simulink model "fkine_test1"  (R2018b)
settings: Solver=FixedStepAuto  StartTime=0.0  StopTime=30  FixedStep=0.01  RelTol=1e-3
InitFcn:
  | runfirst
values from neighbouring files (symbols this model uses):
  bL = 22    [runfirst.m]
  bWb = 15.5    [runfirst.m]
  bWs = 13.5    [runfirst.m]
  d1 = 0    [runfirst.m]
  d2 = 0    [runfirst.m]
  L1 = 3.4    [runfirst.m]
  L2 = 9.5    [runfirst.m]
  L3 = 14.2    [runfirst.m]
settings Model: Creator=skakd  LastModifiedBy=skakd

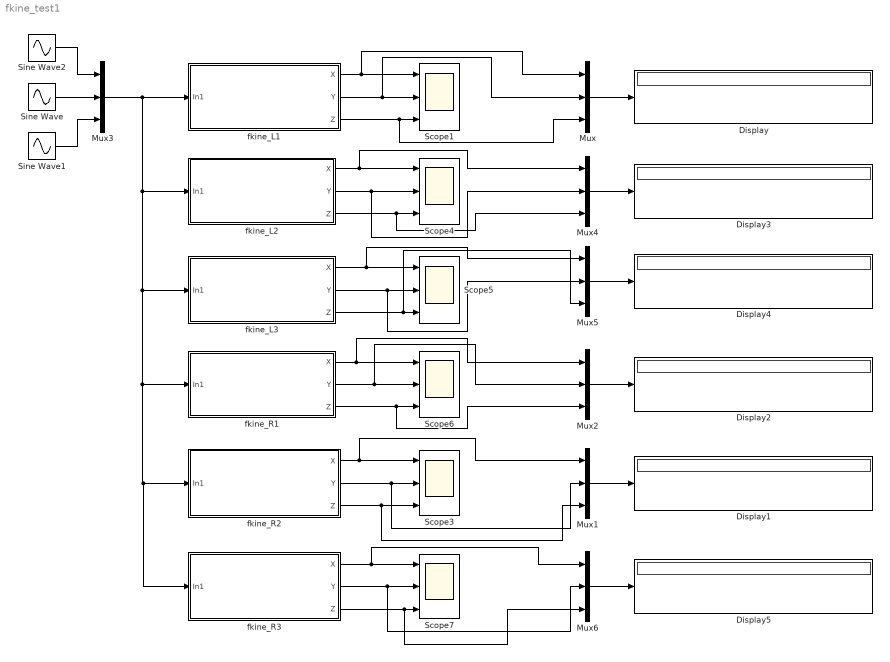
== system fkine_test1 ==
  Display{,1..5} (6 alike) : Display
  Mux{,1..6} (7 alike) : Mux  Inputs=3
  Scope{1,3..7} (6 alike) : Scope  NumInputPorts=3
  Sine Wave : Sin  Amplitude=10  SampleTime=0
  Sine Wave1 : Sin  Amplitude=2.4  Frequency=1.7  SampleTime=0
  Sine Wave2 : Sin  Amplitude=3  Frequency=3.5  SampleTime=0
  fkine_L1 : Subsystem
  fkine_L2 : Subsystem
  fkine_L3 : Subsystem
  fkine_R1 : Subsystem
  fkine_R2 : Subsystem
  fkine_R3 : Subsystem
  wires:
  Sine Wave/1 -> Mux3/2
  Sine Wave1/1 -> Mux3/3
  Sine Wave2/1 -> Mux3/1
  Mux3/1 -> fkine_R3/1(In1), fkine_R2/1(In1), fkine_R1/1(In1), fkine_L3/1(In1), fkine_L2/1(In1), fkine_L1/1(In1)
  fkine_R2/1(X) -> Mux1/1, Scope3/1
  fkine_R2/2(Y) -> Mux1/2, Scope3/2
  fkine_R2/3(Z) -> Mux1/3, Scope3/3
  fkine_L1/1(X) -> Mux/1, Scope1/1
  fkine_L1/2(Y) -> Mux/2, Scope1/2
  fkine_L1/3(Z) -> Mux/3, Scope1/3
  fkine_L2/1(X) -> Mux4/1, Scope4/1
  fkine_L2/2(Y) -> Mux4/2, Scope4/2
  fkine_L2/3(Z) -> Mux4/3, Scope4/3
  fkine_L3/1(X) -> Mux5/1, Scope5/1
  fkine_L3/2(Y) -> Mux5/2, Scope5/2
  fkine_L3/3(Z) -> Mux5/3, Scope5/3
  fkine_R1/1(X) -> Mux2/1, Scope6/1
  fkine_R1/2(Y) -> Mux2/2, Scope6/2
  fkine_R1/3(Z) -> Mux2/3, Scope6/3
  fkine_R3/1(X) -> Mux6/1, Scope7/1
  fkine_R3/2(Y) -> Mux6/2, Scope7/2
  fkine_R3/3(Z) -> Mux6/3, Scope7/3
  Mux/1 -> Display/1
  Mux1/1 -> Display1/1
  Mux2/1 -> Display2/1
  Mux4/1 -> Display3/1
  Mux5/1 -> Display4/1
  Mux6/1 -> Display5/1

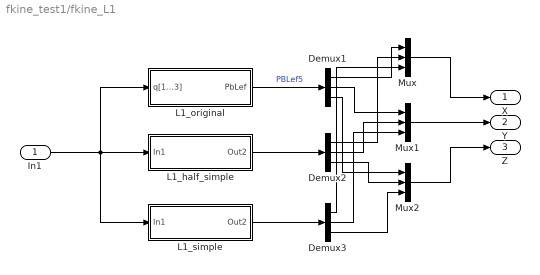
== system fkine_test1/fkine_L1 ==
  In1 : Inport
  Demux1 : Demux  Outputs=3
  Demux2 : Demux  Outputs=3
  Demux3 : Demux  Outputs=3
  L1_half_simple : Subsystem
  L1_original : Subsystem
  L1_simple : Subsystem
  Mux : Mux  Inputs=3
  Mux1 : Mux  Inputs=3
  Mux2 : Mux  Inputs=3
  X : Outport
  Y : Outport  Port=2
  Z : Outport  Port=3
  wires:
  Demux3/2 -> Mux1/3
  L1_original/1(PbLef) -> Demux1/1  "PBLef5"
  Demux3/1 -> Mux/3
  Demux1/1 -> Mux/1
  Demux2/2 -> Mux1/2
  Demux1/3 -> Mux2/1
  Mux2/1 -> Z/1
  Demux1/2 -> Mux1/1
  L1_simple/1(Out2) -> Demux3/1
  Demux2/3 -> Mux2/2
  L1_half_simple/1(Out2) -> Demux2/1
  In1/1 -> L1_simple/1(In1), L1_half_simple/1(In1), L1_original/1(q[1...3])
  Demux2/1 -> Mux/2
  Demux3/3 -> Mux2/3
  Mux/1 -> X/1
  Mux1/1 -> Y/1

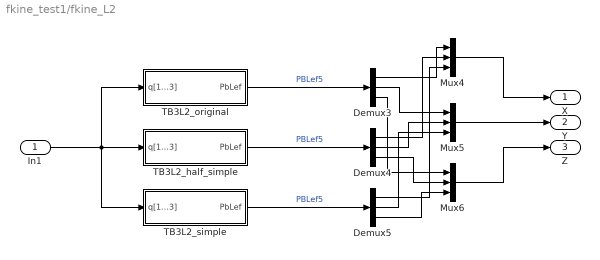
== system fkine_test1/fkine_L2 ==
  In1 : Inport
  Demux3 : Demux  Outputs=3
  Demux4 : Demux  Outputs=3
  Demux5 : Demux  Outputs=3
  Mux4 : Mux  Inputs=3
  Mux5 : Mux  Inputs=3
  Mux6 : Mux  Inputs=3
  TB3L2_half_simple : Subsystem
  TB3L2_original : Subsystem
  TB3L2_simple : Subsystem
  X : Outport
  Y : Outport  Port=2
  Z : Outport  Port=3
  wires:
  Demux4/1 -> Mux4/2
  In1/1 -> TB3L2_half_simple/1(q[1...3]), TB3L2_simple/1(q[1...3]), TB3L2_original/1(q[1...3])
  Demux3/1 -> Mux4/1
  Demux4/2 -> Mux5/2
  TB3L2_half_simple/1(PbLef) -> Demux4/1  "PBLef5"
  Demux5/1 -> Mux4/3
  Demux3/2 -> Mux5/1
  Demux3/3 -> Mux6/1
  Demux5/2 -> Mux5/3
  Demux4/3 -> Mux6/2
  TB3L2_original/1(PbLef) -> Demux3/1  "PBLef5"
  TB3L2_simple/1(PbLef) -> Demux5/1  "PBLef5"
  Demux5/3 -> Mux6/3
  Mux6/1 -> Z/1
  Mux5/1 -> Y/1
  Mux4/1 -> X/1

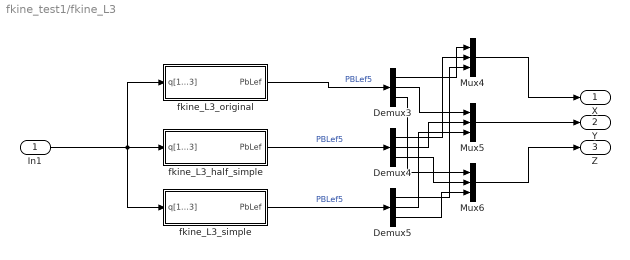
== system fkine_test1/fkine_L3 ==
  In1 : Inport
  Demux3 : Demux  Outputs=3
  Demux4 : Demux  Outputs=3
  Demux5 : Demux  Outputs=3
  Mux4 : Mux  Inputs=3
  Mux5 : Mux  Inputs=3
  Mux6 : Mux  Inputs=3
  fkine_L3_half_simple : Subsystem
  fkine_L3_original : Subsystem
  fkine_L3_simple : Subsystem
  X : Outport
  Y : Outport  Port=2
  Z : Outport  Port=3
  wires:
  Demux3/3 -> Mux6/1
  fkine_L3_original/1(PbLef) -> Demux3/1  "PBLef5"
  In1/1 -> fkine_L3_original/1(q[1...3]), fkine_L3_simple/1(q[1...3]), fkine_L3_half_simple/1(q[1...3])
  Demux3/2 -> Mux5/1
  Demux4/3 -> Mux6/2
  Demux5/1 -> Mux4/3
  fkine_L3_simple/1(PbLef) -> Demux5/1  "PBLef5"
  Demux5/3 -> Mux6/3
  Demux3/1 -> Mux4/1
  Demux5/2 -> Mux5/3
  Mux6/1 -> Z/1
  Demux4/1 -> Mux4/2
  Mux5/1 -> Y/1
  Demux4/2 -> Mux5/2
  Mux4/1 -> X/1
  fkine_L3_half_simple/1(PbLef) -> Demux4/1  "PBLef5"

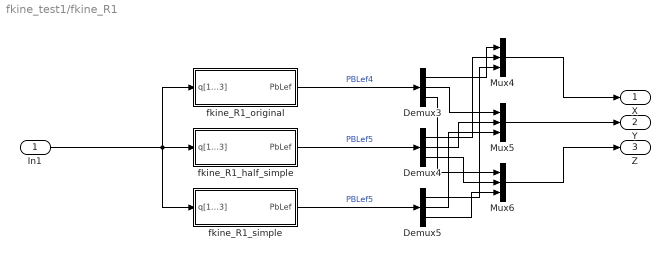
== system fkine_test1/fkine_R1 ==
  In1 : Inport
  Demux3 : Demux  Outputs=3
  Demux4 : Demux  Outputs=3
  Demux5 : Demux  Outputs=3
  Mux4 : Mux  Inputs=3
  Mux5 : Mux  Inputs=3
  Mux6 : Mux  Inputs=3
  fkine_R1_half_simple : Subsystem
  fkine_R1_original : Subsystem
  fkine_R1_simple : Subsystem
  X : Outport
  Y : Outport  Port=2
  Z : Outport  Port=3
  wires:
  Demux3/3 -> Mux6/1
  Demux3/1 -> Mux4/1
  In1/1 -> fkine_R1_simple/1(q[1...3]), fkine_R1_original/1(q[1...3]), fkine_R1_half_simple/1(q[1...3])
  fkine_R1_half_simple/1(PbLef) -> Demux4/1  "PBLef5"
  fkine_R1_simple/1(PbLef) -> Demux5/1  "PBLef5"
  Demux4/1 -> Mux4/2
  Demux5/3 -> Mux6/3
  Demux5/2 -> Mux5/3
  Demux5/1 -> Mux4/3
  Demux4/3 -> Mux6/2
  Demux3/2 -> Mux5/1
  Mux4/1 -> X/1
  Demux4/2 -> Mux5/2
  fkine_R1_original/1(PbLef) -> Demux3/1  "PBLef4"
  Mux6/1 -> Z/1
  Mux5/1 -> Y/1

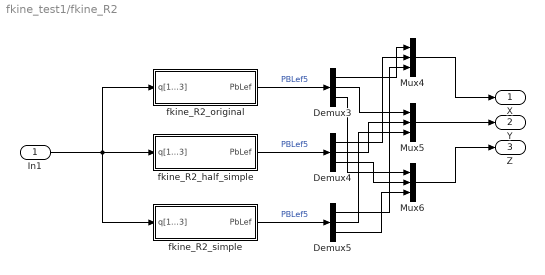
== system fkine_test1/fkine_R2 ==
  In1 : Inport
  Demux3 : Demux  Outputs=3
  Demux4 : Demux  Outputs=3
  Demux5 : Demux  Outputs=3
  Mux4 : Mux  Inputs=3
  Mux5 : Mux  Inputs=3
  Mux6 : Mux  Inputs=3
  fkine_R2_half_simple : Subsystem
  fkine_R2_original : Subsystem
  fkine_R2_simple : Subsystem
  X : Outport
  Y : Outport  Port=2
  Z : Outport  Port=3
  wires:
  Demux3/2 -> Mux5/1
  fkine_R2_half_simple/1(PbLef) -> Demux4/1  "PBLef5"
  Demux4/1 -> Mux4/2
  In1/1 -> fkine_R2_half_simple/1(q[1...3]), fkine_R2_simple/1(q[1...3]), fkine_R2_original/1(q[1...3])
  Demux4/2 -> Mux5/2
  fkine_R2_simple/1(PbLef) -> Demux5/1  "PBLef5"
  Demux5/1 -> Mux4/3
  Demux5/2 -> Mux5/3
  Demux5/3 -> Mux6/3
  Demux3/1 -> Mux4/1
  Demux3/3 -> Mux6/1
  Demux4/3 -> Mux6/2
  fkine_R2_original/1(PbLef) -> Demux3/1  "PBLef5"
  Mux6/1 -> Z/1
  Mux4/1 -> X/1
  Mux5/1 -> Y/1

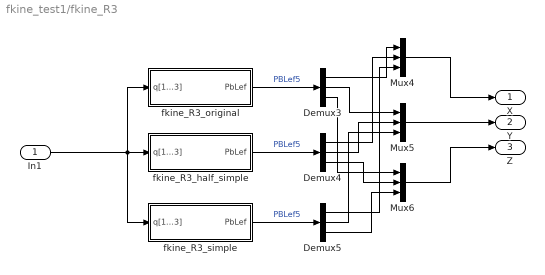
== system fkine_test1/fkine_R3 ==
  In1 : Inport
  Demux3 : Demux  Outputs=3
  Demux4 : Demux  Outputs=3
  Demux5 : Demux  Outputs=3
  Mux4 : Mux  Inputs=3
  Mux5 : Mux  Inputs=3
  Mux6 : Mux  Inputs=3
  fkine_R3_half_simple : Subsystem
  fkine_R3_original : Subsystem
  fkine_R3_simple : Subsystem
  X : Outport
  Y : Outport  Port=2
  Z : Outport  Port=3
  wires:
  Demux4/3 -> Mux6/2
  In1/1 -> fkine_R3_original/1(q[1...3]), fkine_R3_simple/1(q[1...3]), fkine_R3_half_simple/1(q[1...3])
  Demux3/3 -> Mux6/1
  fkine_R3_simple/1(PbLef) -> Demux5/1  "PBLef5"
  fkine_R3_original/1(PbLef) -> Demux3/1  "PBLef5"
  Demux4/1 -> Mux4/2
  Demux3/1 -> Mux4/1
  Demux5/2 -> Mux5/3
  Mux6/1 -> Z/1
  Demux4/2 -> Mux5/2
  Demux5/3 -> Mux6/3
  Demux5/1 -> Mux4/3
  Demux3/2 -> Mux5/1
  fkine_R3_half_simple/1(PbLef) -> Demux4/1  "PBLef5"
  Mux4/1 -> X/1
  Mux5/1 -> Y/1

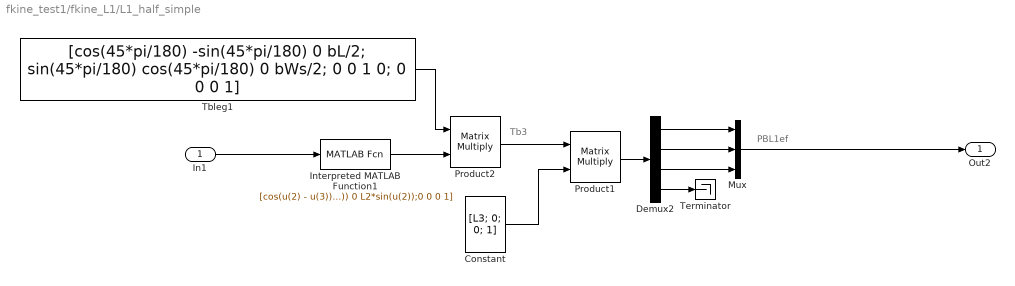
== system fkine_test1/fkine_L1/L1_half_simple ==
  note: Tb3
  note: PBL1ef
  In1 : Inport
  Constant : Constant  Value=[L3; 0; 0; 1]  VectorParams1D=off
  Demux2 : Demux
  Interpreted MATLAB Function1 : MATLABFcn  MATLABFcn=[cos(u(2) - u(3))*cos(u(1)) sin(u(2) - u(3))*cos(u(1)) -sin(u(1)) cos(u(1))*(L1 + L2*cos(u(2))); cos(u(2) - u(3))*sin(u(1)) sin(u(2) - u(3))*sin(u(1)) cos(u(1)) sin(u(1))*(L1 + L2*cos(u(2))); sin(u(2) - u(3)) -cos(u(2) - u(3)) 0 L2*sin(u(2));0 0 0 1]  Output1D=off
  Mux : Mux  Inputs=3
  Product1 : Product  Multiplication=Matrix(*)
  Product2 : Product  Multiplication=Matrix(*)
  Tbleg1 : Constant  Value=[cos(45*pi/180) -sin(45*pi/180) 0 bL/2; sin(45*pi/180) cos(45*pi/180) 0 bWs/2; 0 0 1 0; 0 0 0 1]  VectorParams1D=off
  Terminator : Terminator
  Out2 : Outport
  wires:
  Demux2/1 -> Mux/1
  Product2/1 -> Product1/1
  Interpreted MATLAB Function1/1 -> Product2/2
  Product1/1 -> Demux2/1
  Constant/1 -> Product1/2
  Demux2/4 -> Terminator/1
  Demux2/2 -> Mux/2
  Tbleg1/1 -> Product2/1
  Demux2/3 -> Mux/3
  Mux/1 -> Out2/1
  In1/1 -> Interpreted MATLAB Function1/1

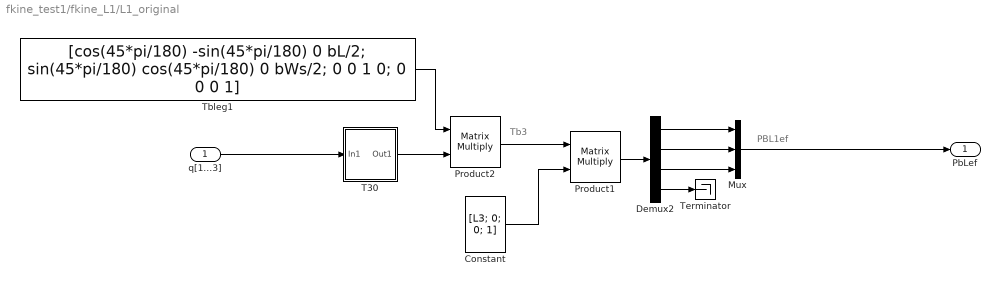
== system fkine_test1/fkine_L1/L1_original ==
  note: PBL1ef
  note: Tb3
  q[1...3] : Inport
  Constant : Constant  Value=[L3; 0; 0; 1]  VectorParams1D=off
  Demux2 : Demux
  Mux : Mux  Inputs=3
  Product1 : Product  Multiplication=Matrix(*)
  Product2 : Product  Multiplication=Matrix(*)
  T30 : Subsystem
  Tbleg1 : Constant  Value=[cos(45*pi/180) -sin(45*pi/180) 0 bL/2; sin(45*pi/180) cos(45*pi/180) 0 bWs/2; 0 0 1 0; 0 0 0 1]  VectorParams1D=off
  Terminator : Terminator
  PbLef : Outport
  wires:
  Product2/1 -> Product1/1
  Demux2/2 -> Mux/2
  Mux/1 -> PbLef/1
  Demux2/1 -> Mux/1
  Demux2/4 -> Terminator/1
  Product1/1 -> Demux2/1
  Demux2/3 -> Mux/3
  Tbleg1/1 -> Product2/1
  T30/1(Out1) -> Product2/2
  q[1...3]/1 -> T30/1(In1)
  Constant/1 -> Product1/2

== system fkine_test1/fkine_L1/L1_simple ==
  note: PBL1ef
  In1 : Inport
  Demux2 : Demux
  Interpreted MATLAB Function1 : MATLABFcn  MATLABFcn=[bL/2 + L3*((2^(1/2)*cos(u(2) - u(3))*cos(u(1)))/2 - (2^(1/2)*cos(u(2) - u(3))*sin(u(1)))/2) + (2^(1/2)*cos(u(1))*(L1 + L2*cos(u(2))))/2 - (2^(1/2)*sin(u(1))*(L1 + L2*cos(u(2))))/2; bWs/2 + L3*((2^(1/2)*cos(u(2) - u(3))*cos(u(1)))/2 + (2^(1/2)*cos(u(2) - u(3))*sin(u(1)))/2) + (2^(1/2)*cos(u(1))*(L1 + L2*cos(u(2))))/2 + (2^(1/2)*sin(u(1))*(L1 + L2*cos(u(2))))/2; L2*sin(u(2)) + L3*sin(u(2) - u(3));1]  Output1D=off
  Mux : Mux  Inputs=3
  Terminator : Terminator
  Out2 : Outport
  wires:
  Demux2/1 -> Mux/1
  Interpreted MATLAB Function1/1 -> Demux2/1
  Demux2/4 -> Terminator/1
  Demux2/2 -> Mux/2
  Demux2/3 -> Mux/3
  Mux/1 -> Out2/1
  In1/1 -> Interpreted MATLAB Function1/1

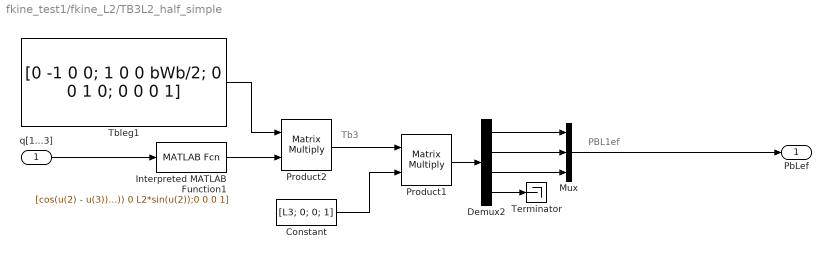
== system fkine_test1/fkine_L2/TB3L2_half_simple ==
  note: Tb3
  note: PBL1ef
  q[1...3] : Inport
  Constant : Constant  Value=[L3; 0; 0; 1]  VectorParams1D=off
  Demux2 : Demux
  Interpreted MATLAB Function1 : MATLABFcn  MATLABFcn=[cos(u(2) - u(3))*cos(u(1)) sin(u(2) - u(3))*cos(u(1)) -sin(u(1)) cos(u(1))*(L1 + L2*cos(u(2))); cos(u(2) - u(3))*sin(u(1)) sin(u(2) - u(3))*sin(u(1)) cos(u(1)) sin(u(1))*(L1 + L2*cos(u(2))); sin(u(2) - u(3)) -cos(u(2) - u(3)) 0 L2*sin(u(2));0 0 0 1]  Output1D=off
  Mux : Mux  Inputs=3
  Product1 : Product  Multiplication=Matrix(*)
  Product2 : Product  Multiplication=Matrix(*)
  Tbleg1 : Constant  Value=[0 -1 0 0; 1 0 0 bWb/2; 0 0 1 0; 0 0 0 1]  VectorParams1D=off
  Terminator : Terminator
  PbLef : Outport
  wires:
  Constant/1 -> Product1/2
  q[1...3]/1 -> Interpreted MATLAB Function1/1
  Interpreted MATLAB Function1/1 -> Product2/2
  Tbleg1/1 -> Product2/1
  Demux2/3 -> Mux/3
  Product1/1 -> Demux2/1
  Demux2/4 -> Terminator/1
  Demux2/1 -> Mux/1
  Mux/1 -> PbLef/1
  Demux2/2 -> Mux/2
  Product2/1 -> Product1/1

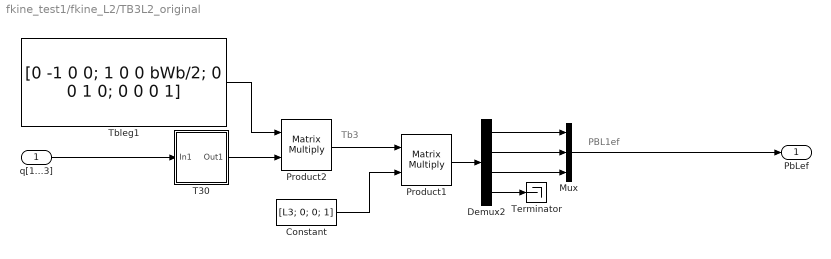
== system fkine_test1/fkine_L2/TB3L2_original ==
  note: Tb3
  note: PBL1ef
  q[1...3] : Inport
  Constant : Constant  Value=[L3; 0; 0; 1]  VectorParams1D=off
  Demux2 : Demux
  Mux : Mux  Inputs=3
  Product1 : Product  Multiplication=Matrix(*)
  Product2 : Product  Multiplication=Matrix(*)
  T30 : Subsystem
  Tbleg1 : Constant  Value=[0 -1 0 0; 1 0 0 bWb/2; 0 0 1 0; 0 0 0 1]  VectorParams1D=off
  Terminator : Terminator
  PbLef : Outport
  wires:
  Constant/1 -> Product1/2
  q[1...3]/1 -> T30/1(In1)
  T30/1(Out1) -> Product2/2
  Tbleg1/1 -> Product2/1
  Demux2/3 -> Mux/3
  Product1/1 -> Demux2/1
  Demux2/4 -> Terminator/1
  Demux2/1 -> Mux/1
  Mux/1 -> PbLef/1
  Demux2/2 -> Mux/2
  Product2/1 -> Product1/1

== system fkine_test1/fkine_L2/TB3L2_simple ==
  note: PBL1ef
  q[1...3] : Inport
  Demux2 : Demux
  Interpreted MATLAB Function2 : MATLABFcn  MATLABFcn=[-sin(u(1))*(L1 + L2*cos(u(2))) - L3*cos(u(2) - u(3))*sin(u(1)); bWb/2 + cos(u(1))*(L1 + L2*cos(u(2))) + L3*cos(u(2) - u(3))*cos(u(1));L2*sin(u(2))+L3*sin(u(2)-u(3));1]  Output1D=off
  Mux : Mux  Inputs=3
  Terminator : Terminator
  PbLef : Outport
  wires:
  Demux2/2 -> Mux/2
  Mux/1 -> PbLef/1
  Demux2/1 -> Mux/1
  Demux2/4 -> Terminator/1
  Interpreted MATLAB Function2/1 -> Demux2/1
  Demux2/3 -> Mux/3
  q[1...3]/1 -> Interpreted MATLAB Function2/1

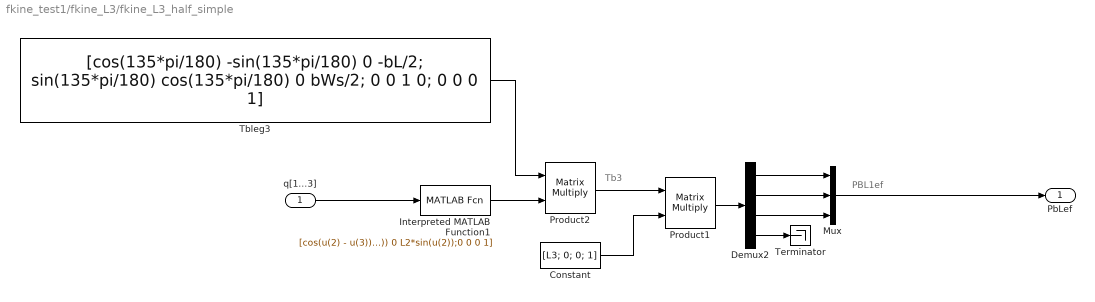
== system fkine_test1/fkine_L3/fkine_L3_half_simple ==
  note: PBL1ef
  note: Tb3
  q[1...3] : Inport
  Constant : Constant  Value=[L3; 0; 0; 1]  VectorParams1D=off
  Demux2 : Demux
  Interpreted MATLAB Function1 : MATLABFcn  MATLABFcn=[cos(u(2) - u(3))*cos(u(1)) sin(u(2) - u(3))*cos(u(1)) -sin(u(1)) cos(u(1))*(L1 + L2*cos(u(2))); cos(u(2) - u(3))*sin(u(1)) sin(u(2) - u(3))*sin(u(1)) cos(u(1)) sin(u(1))*(L1 + L2*cos(u(2))); sin(u(2) - u(3)) -cos(u(2) - u(3)) 0 L2*sin(u(2));0 0 0 1]  Output1D=off
  Mux : Mux  Inputs=3
  Product1 : Product  Multiplication=Matrix(*)
  Product2 : Product  Multiplication=Matrix(*)
  Tbleg3 : Constant  Value=[cos(135*pi/180) -sin(135*pi/180) 0 -bL/2; sin(135*pi/180) cos(135*pi/180) 0 bWs/2; 0 0 1 0; 0 0 0 1]  VectorParams1D=off
  Terminator : Terminator
  PbLef : Outport
  wires:
  Product2/1 -> Product1/1
  Demux2/2 -> Mux/2
  Mux/1 -> PbLef/1
  Demux2/1 -> Mux/1
  Demux2/4 -> Terminator/1
  Product1/1 -> Demux2/1
  Demux2/3 -> Mux/3
  Tbleg3/1 -> Product2/1
  Interpreted MATLAB Function1/1 -> Product2/2
  q[1...3]/1 -> Interpreted MATLAB Function1/1
  Constant/1 -> Product1/2

== system fkine_test1/fkine_L3/fkine_L3_original ==
  note: PBL1ef
  note: Tb3
  q[1...3] : Inport
  Constant : Constant  Value=[L3; 0; 0; 1]  VectorParams1D=off
  Demux2 : Demux
  Mux : Mux  Inputs=3
  Product1 : Product  Multiplication=Matrix(*)
  Product2 : Product  Multiplication=Matrix(*)
  T30 : Subsystem
  Tbleg3 : Constant  Value=[cos(135*pi/180) -sin(135*pi/180) 0 -bL/2; sin(135*pi/180) cos(135*pi/180) 0 bWs/2; 0 0 1 0; 0 0 0 1]  VectorParams1D=off
  Terminator : Terminator
  PbLef : Outport
  wires:
  Product2/1 -> Product1/1
  Demux2/2 -> Mux/2
  Mux/1 -> PbLef/1
  Demux2/1 -> Mux/1
  Demux2/4 -> Terminator/1
  Product1/1 -> Demux2/1
  Demux2/3 -> Mux/3
  Tbleg3/1 -> Product2/1
  T30/1(Out1) -> Product2/2
  q[1...3]/1 -> T30/1(In1)
  Constant/1 -> Product1/2

== system fkine_test1/fkine_L3/fkine_L3_simple ==
  note: PBL1ef
  q[1...3] : Inport
  Demux2 : Demux
  Interpreted MATLAB Function1 : MATLABFcn  MATLABFcn=[-bL/2-L3*((2^(1/2)*cos(u(2)-u(3))*cos(u(1)))/2+(2^(1/2)*cos(u(2)-u(3))*sin(u(1)))/2)-(2^(1/2)*cos(u(1))*(L1+L2*cos(u(2))))/2 - (2^(1/2)*sin(u(1))*(L1 + L2*cos(u(2))))/2; bWs/2 + L3*((2^(1/2)*cos(u(2)-u(3))*cos(u(1)))/2-(2^(1/2)*cos(u(2)-u(3))*sin(u(1)))/2)+(2^(1/2)*cos(u(1))*(L1+L2*cos(u(2))))/2-(2^(1/2)*sin(u(1))*(L1+L2*cos(u(2))))/2; L2*sin(u(2))+L3*sin(u(2)-u(3)); 1]  Output1D=off
  Mux : Mux  Inputs=3
  Terminator : Terminator
  PbLef : Outport
  wires:
  q[1...3]/1 -> Interpreted MATLAB Function1/1
  Demux2/3 -> Mux/3
  Interpreted MATLAB Function1/1 -> Demux2/1
  Demux2/4 -> Terminator/1
  Demux2/1 -> Mux/1
  Mux/1 -> PbLef/1
  Demux2/2 -> Mux/2

== system fkine_test1/fkine_R1/fkine_R1_half_simple ==
  note: PBL1ef
  note: Tb3
  q[1...3] : Inport
  Constant : Constant  Value=[L3; 0; 0; 1]  VectorParams1D=off
  Demux2 : Demux
  Interpreted MATLAB Function1 : MATLABFcn  MATLABFcn=[cos(u(2) - u(3))*cos(u(1)) sin(u(2) - u(3))*cos(u(1)) -sin(u(1)) cos(u(1))*(L1 + L2*cos(u(2))); cos(u(2) - u(3))*sin(u(1)) sin(u(2) - u(3))*sin(u(1)) cos(u(1)) sin(u(1))*(L1 + L2*cos(u(2))); sin(u(2) - u(3)) -cos(u(2) - u(3)) 0 L2*sin(u(2));0 0 0 1]  Output1D=off
  Mux : Mux  Inputs=3
  Product1 : Product  Multiplication=Matrix(*)
  Product2 : Product  Multiplication=Matrix(*)
  Tbleg1 : Constant  Value=[cos(-45*pi/180) -sin(-45*pi/180) 0 bL/2; sin(-45*pi/180) cos(-45*pi/180) 0 -bWs/2; 0 0 1 0; 0 0 0 1]  VectorParams1D=off
  Terminator : Terminator
  PbLef : Outport
  wires:
  Product2/1 -> Product1/1
  Demux2/2 -> Mux/2
  Mux/1 -> PbLef/1
  Demux2/1 -> Mux/1
  Demux2/4 -> Terminator/1
  Product1/1 -> Demux2/1
  Demux2/3 -> Mux/3
  Tbleg1/1 -> Product2/1
  Interpreted MATLAB Function1/1 -> Product2/2
  q[1...3]/1 -> Interpreted MATLAB Function1/1
  Constant/1 -> Product1/2

== system fkine_test1/fkine_R1/fkine_R1_original ==
  note: Tb3
  note: PBL1ef
  q[1...3] : Inport
  Constant : Constant  Value=[L3; 0; 0; 1]  VectorParams1D=off
  Demux2 : Demux
  Mux : Mux  Inputs=3
  Product1 : Product  Multiplication=Matrix(*)
  Product2 : Product  Multiplication=Matrix(*)
  T30 : Subsystem
  Tbleg1 : Constant  Value=[cos(-45*pi/180) -sin(-45*pi/180) 0 bL/2; sin(-45*pi/180) cos(-45*pi/180) 0 -bWs/2; 0 0 1 0; 0 0 0 1]  VectorParams1D=off
  Terminator : Terminator
  PbLef : Outport
  wires:
  Constant/1 -> Product1/2
  q[1...3]/1 -> T30/1(In1)
  T30/1(Out1) -> Product2/2
  Tbleg1/1 -> Product2/1
  Demux2/3 -> Mux/3
  Product1/1 -> Demux2/1
  Demux2/4 -> Terminator/1
  Demux2/1 -> Mux/1
  Mux/1 -> PbLef/1
  Demux2/2 -> Mux/2
  Product2/1 -> Product1/1

== system fkine_test1/fkine_R1/fkine_R1_simple ==
  note: PBL1ef
  q[1...3] : Inport
  Demux2 : Demux
  Interpreted MATLAB Function1 : MATLABFcn  MATLABFcn=[bL/2 + L3*((2^(1/2)*cos(u(2) - u(3))*cos(u(1)))/2 + (2^(1/2)*cos(u(2) - u(3))*sin(u(1)))/2) + (2^(1/2)*cos(u(1))*(L1 + L2*cos(u(2))))/2 + (2^(1/2)*sin(u(1))*(L1 + L2*cos(u(2))))/2; (2^(1/2)*sin(u(1))*(L1 + L2*cos(u(2))))/2 - L3*((2^(1/2)*cos(u(2) - u(3))*cos(u(1)))/2 - (2^(1/2)*cos(u(2) - u(3))*sin(u(1)))/2) - (2^(1/2)*cos(u(1))*(L1 + L2*cos(u(2))))/2 - bWs/2;L2*sin(u(2)) + L3*sin(u(2) - u(3));1]  Output1D=off
  Mux : Mux  Inputs=3
  Terminator : Terminator
  PbLef : Outport
  wires:
  q[1...3]/1 -> Interpreted MATLAB Function1/1
  Demux2/3 -> Mux/3
  Interpreted MATLAB Function1/1 -> Demux2/1
  Demux2/4 -> Terminator/1
  Demux2/1 -> Mux/1
  Mux/1 -> PbLef/1
  Demux2/2 -> Mux/2

== system fkine_test1/fkine_R2/fkine_R2_half_simple ==
  note: PBL1ef
  note: Tb3
  q[1...3] : Inport
  Constant : Constant  Value=[L3; 0; 0; 1]  VectorParams1D=off
  Demux2 : Demux
  Interpreted MATLAB Function1 : MATLABFcn  MATLABFcn=[cos(u(2) - u(3))*cos(u(1)) sin(u(2) - u(3))*cos(u(1)) -sin(u(1)) cos(u(1))*(L1 + L2*cos(u(2))); cos(u(2) - u(3))*sin(u(1)) sin(u(2) - u(3))*sin(u(1)) cos(u(1)) sin(u(1))*(L1 + L2*cos(u(2))); sin(u(2) - u(3)) -cos(u(2) - u(3)) 0 L2*sin(u(2));0 0 0 1]  Output1D=off
  Mux : Mux  Inputs=3
  Product1 : Product  Multiplication=Matrix(*)
  Product2 : Product  Multiplication=Matrix(*)
  Tbleg1 : Constant  Value=[0 1 0 0; -1 0 0 -bWb/2; 0 0 1 0; 0 0 0 1]  VectorParams1D=off
  Terminator : Terminator
  PbLef : Outport
  wires:
  Product2/1 -> Product1/1
  Demux2/2 -> Mux/2
  Mux/1 -> PbLef/1
  Demux2/1 -> Mux/1
  Demux2/4 -> Terminator/1
  Product1/1 -> Demux2/1
  Demux2/3 -> Mux/3
  Tbleg1/1 -> Product2/1
  Interpreted MATLAB Function1/1 -> Product2/2
  q[1...3]/1 -> Interpreted MATLAB Function1/1
  Constant/1 -> Product1/2

== system fkine_test1/fkine_R2/fkine_R2_original ==
  note: PBL1ef
  note: Tb3
  q[1...3] : Inport
  Constant : Constant  Value=[L3; 0; 0; 1]  VectorParams1D=off
  Demux2 : Demux
  Mux : Mux  Inputs=3
  Product1 : Product  Multiplication=Matrix(*)
  Product2 : Product  Multiplication=Matrix(*)
  T30 : Subsystem
  Tbleg1 : Constant  Value=[0 1 0 0; -1 0 0 -bWb/2; 0 0 1 0; 0 0 0 1]  VectorParams1D=off
  Terminator : Terminator
  PbLef : Outport
  wires:
  Product2/1 -> Product1/1
  Demux2/2 -> Mux/2
  Mux/1 -> PbLef/1
  Demux2/1 -> Mux/1
  Demux2/4 -> Terminator/1
  Product1/1 -> Demux2/1
  Demux2/3 -> Mux/3
  Tbleg1/1 -> Product2/1
  T30/1(Out1) -> Product2/2
  q[1...3]/1 -> T30/1(In1)
  Constant/1 -> Product1/2

== system fkine_test1/fkine_R2/fkine_R2_simple ==
  note: PBL1ef
  q[1...3] : Inport
  Demux2 : Demux
  Interpreted MATLAB Function1 : MATLABFcn  MATLABFcn=[sin(u(1))*(L1+L2*cos(u(2)))+L3*cos(u(2)-u(3))*sin(u(1)); -bWb/2-cos(u(1))*(L1+L2*cos(u(2)))-L3*cos(u(2)-u(3))*cos(u(1)); L2*sin(u(2))+L3*sin(u(2)-u(3));1]  Output1D=off
  Mux : Mux  Inputs=3
  Terminator : Terminator
  PbLef : Outport
  wires:
  q[1...3]/1 -> Interpreted MATLAB Function1/1
  Demux2/3 -> Mux/3
  Interpreted MATLAB Function1/1 -> Demux2/1
  Demux2/4 -> Terminator/1
  Demux2/1 -> Mux/1
  Mux/1 -> PbLef/1
  Demux2/2 -> Mux/2

== system fkine_test1/fkine_R3/fkine_R3_half_simple ==
  note: Tb3
  note: PBL1ef
  q[1...3] : Inport
  Constant : Constant  Value=[L3; 0; 0; 1]  VectorParams1D=off
  Demux2 : Demux
  Interpreted MATLAB Function1 : MATLABFcn  MATLABFcn=[cos(u(2) - u(3))*cos(u(1)) sin(u(2) - u(3))*cos(u(1)) -sin(u(1)) cos(u(1))*(L1 + L2*cos(u(2))); cos(u(2) - u(3))*sin(u(1)) sin(u(2) - u(3))*sin(u(1)) cos(u(1)) sin(u(1))*(L1 + L2*cos(u(2))); sin(u(2) - u(3)) -cos(u(2) - u(3)) 0 L2*sin(u(2));0 0 0 1]  Output1D=off
  Mux : Mux  Inputs=3
  Product1 : Product  Multiplication=Matrix(*)
  Product2 : Product  Multiplication=Matrix(*)
  Tbleg1 : Constant  Value=[cos(-135*pi/180) -sin(-135*pi/180) 0 -bL/2; sin(-135*pi/180) cos(-135*pi/180) 0 -bWs/2; 0 0 1 0; 0 0 0 1]  VectorParams1D=off
  Terminator : Terminator
  PbLef : Outport
  wires:
  Constant/1 -> Product1/2
  q[1...3]/1 -> Interpreted MATLAB Function1/1
  Interpreted MATLAB Function1/1 -> Product2/2
  Tbleg1/1 -> Product2/1
  Demux2/3 -> Mux/3
  Product1/1 -> Demux2/1
  Demux2/4 -> Terminator/1
  Demux2/1 -> Mux/1
  Mux/1 -> PbLef/1
  Demux2/2 -> Mux/2
  Product2/1 -> Product1/1

== system fkine_test1/fkine_R3/fkine_R3_original ==
  note: PBL1ef
  note: Tb3
  q[1...3] : Inport
  Constant : Constant  Value=[L3; 0; 0; 1]  VectorParams1D=off
  Demux2 : Demux
  Mux : Mux  Inputs=3
  Product1 : Product  Multiplication=Matrix(*)
  Product2 : Product  Multiplication=Matrix(*)
  T30 : Subsystem
  Tbleg1 : Constant  Value=[cos(-135*pi/180) -sin(-135*pi/180) 0 -bL/2; sin(-135*pi/180) cos(-135*pi/180) 0 -bWs/2; 0 0 1 0; 0 0 0 1]  VectorParams1D=off
  Terminator : Terminator
  PbLef : Outport
  wires:
  Product2/1 -> Product1/1
  Demux2/2 -> Mux/2
  Mux/1 -> PbLef/1
  Demux2/1 -> Mux/1
  Demux2/4 -> Terminator/1
  Product1/1 -> Demux2/1
  Demux2/3 -> Mux/3
  Tbleg1/1 -> Product2/1
  T30/1(Out1) -> Product2/2
  q[1...3]/1 -> T30/1(In1)
  Constant/1 -> Product1/2

== system fkine_test1/fkine_R3/fkine_R3_simple ==
  note: PBL1ef
  q[1...3] : Inport
  Demux2 : Demux
  Interpreted MATLAB Function1 : MATLABFcn  MATLABFcn=[(2^(1/2)*sin(u(1))*(L1 + L2*cos(u(2))))/2 - L3*((2^(1/2)*cos(u(2) - u(3))*cos(u(1)))/2 - (2^(1/2)*cos(u(2) - u(3))*sin(u(1)))/2) - (2^(1/2)*cos(u(1))*(L1 + L2*cos(u(2))))/2 - bL/2; -bWs/2-L3*((2^(1/2)*cos(u(2)-u(3))*cos(u(1)))/2 + (2^(1/2)*cos(u(2) - u(3))*sin(u(1)))/2) - (2^(1/2)*cos(u(1))*(L1 + L2*cos(u(2))))/2 - (2^(1/2)*sin(u(1))*(L1 + L2*cos(u(2))))/2; L2*sin(u(2)) + L3*sin(u(2) - u(3)); 1]  Output1D=off
  Mux : Mux  Inputs=3
  Terminator : Terminator
  PbLef : Outport
  wires:
  Demux2/2 -> Mux/2
  Mux/1 -> PbLef/1
  Demux2/1 -> Mux/1
  Demux2/4 -> Terminator/1
  Interpreted MATLAB Function1/1 -> Demux2/1
  Demux2/3 -> Mux/3
  q[1...3]/1 -> Interpreted MATLAB Function1/1

== system fkine_test1/fkine_L1/L1_original/T30 ==
  In1 : Inport
  Demux1 : Demux  Outputs=3
  Interpreted MATLAB Function : MATLABFcn  MATLABFcn=[cos(u) -sin(u) 0 0; sin(u) cos(u) 0 0; 0 0 1 d1; 0 0 0 1]  Output1D=off
  Interpreted MATLAB Function1 : MATLABFcn  MATLABFcn=[cos(u) -sin(u) 0 L1; 0 0 -1 0; sin(u) cos(u) 0 -abs(d2); 0 0 0 1]  Output1D=off
  Interpreted MATLAB Function2 : MATLABFcn  MATLABFcn=[cos(u) -sin(u) 0 L2; -sin(u) -cos(u) 0 0; 0 0 -1 0; 0 0 0 1]  Output1D=off
  Product : Product  Inputs=3  Multiplication=Matrix(*)
  Out1 : Outport
  wires:
  Demux1/1 -> Interpreted MATLAB Function/1
  In1/1 -> Demux1/1
  Product/1 -> Out1/1
  Demux1/2 -> Interpreted MATLAB Function1/1
  Demux1/3 -> Interpreted MATLAB Function2/1
  Interpreted MATLAB Function/1 -> Product/1
  Interpreted MATLAB Function1/1 -> Product/2
  Interpreted MATLAB Function2/1 -> Product/3

== system fkine_test1/fkine_L2/TB3L2_original/T30 ==
  In1 : Inport
  Demux1 : Demux  Outputs=3
  Interpreted MATLAB Function : MATLABFcn  MATLABFcn=[cos(u) -sin(u) 0 0; sin(u) cos(u) 0 0; 0 0 1 d1; 0 0 0 1]  Output1D=off
  Interpreted MATLAB Function1 : MATLABFcn  MATLABFcn=[cos(u) -sin(u) 0 L1; 0 0 -1 0; sin(u) cos(u) 0 -abs(d2); 0 0 0 1]  Output1D=off
  Interpreted MATLAB Function2 : MATLABFcn  MATLABFcn=[cos(u) -sin(u) 0 L2; -sin(u) -cos(u) 0 0; 0 0 -1 0; 0 0 0 1]  Output1D=off
  Product : Product  Inputs=3  Multiplication=Matrix(*)
  Out1 : Outport
  wires:
  Demux1/1 -> Interpreted MATLAB Function/1
  In1/1 -> Demux1/1
  Product/1 -> Out1/1
  Demux1/2 -> Interpreted MATLAB Function1/1
  Demux1/3 -> Interpreted MATLAB Function2/1
  Interpreted MATLAB Function/1 -> Product/1
  Interpreted MATLAB Function1/1 -> Product/2
  Interpreted MATLAB Function2/1 -> Product/3

== system fkine_test1/fkine_L3/fkine_L3_original/T30 ==
  In1 : Inport
  Demux1 : Demux  Outputs=3
  Interpreted MATLAB Function : MATLABFcn  MATLABFcn=[cos(u) -sin(u) 0 0; sin(u) cos(u) 0 0; 0 0 1 d1; 0 0 0 1]  Output1D=off
  Interpreted MATLAB Function1 : MATLABFcn  MATLABFcn=[cos(u) -sin(u) 0 L1; 0 0 -1 0; sin(u) cos(u) 0 -abs(d2); 0 0 0 1]  Output1D=off
  Interpreted MATLAB Function2 : MATLABFcn  MATLABFcn=[cos(u) -sin(u) 0 L2; -sin(u) -cos(u) 0 0; 0 0 -1 0; 0 0 0 1]  Output1D=off
  Product : Product  Inputs=3  Multiplication=Matrix(*)
  Out1 : Outport
  wires:
  Demux1/1 -> Interpreted MATLAB Function/1
  In1/1 -> Demux1/1
  Product/1 -> Out1/1
  Demux1/2 -> Interpreted MATLAB Function1/1
  Demux1/3 -> Interpreted MATLAB Function2/1
  Interpreted MATLAB Function/1 -> Product/1
  Interpreted MATLAB Function1/1 -> Product/2
  Interpreted MATLAB Function2/1 -> Product/3

== system fkine_test1/fkine_R1/fkine_R1_original/T30 ==
  In1 : Inport
  Demux1 : Demux  Outputs=3
  Interpreted MATLAB Function : MATLABFcn  MATLABFcn=[cos(u) -sin(u) 0 0; sin(u) cos(u) 0 0; 0 0 1 d1; 0 0 0 1]  Output1D=off
  Interpreted MATLAB Function1 : MATLABFcn  MATLABFcn=[cos(u) -sin(u) 0 L1; 0 0 -1 0; sin(u) cos(u) 0 -abs(d2); 0 0 0 1]  Output1D=off
  Interpreted MATLAB Function2 : MATLABFcn  MATLABFcn=[cos(u) -sin(u) 0 L2; -sin(u) -cos(u) 0 0; 0 0 -1 0; 0 0 0 1]  Output1D=off
  Product : Product  Inputs=3  Multiplication=Matrix(*)
  Out1 : Outport
  wires:
  Demux1/1 -> Interpreted MATLAB Function/1
  In1/1 -> Demux1/1
  Product/1 -> Out1/1
  Demux1/2 -> Interpreted MATLAB Function1/1
  Demux1/3 -> Interpreted MATLAB Function2/1
  Interpreted MATLAB Function/1 -> Product/1
  Interpreted MATLAB Function1/1 -> Product/2
  Interpreted MATLAB Function2/1 -> Product/3

== system fkine_test1/fkine_R2/fkine_R2_original/T30 ==
  In1 : Inport
  Demux1 : Demux  Outputs=3
  Interpreted MATLAB Function : MATLABFcn  MATLABFcn=[cos(u) -sin(u) 0 0; sin(u) cos(u) 0 0; 0 0 1 d1; 0 0 0 1]  Output1D=off
  Interpreted MATLAB Function1 : MATLABFcn  MATLABFcn=[cos(u) -sin(u) 0 L1; 0 0 -1 0; sin(u) cos(u) 0 -abs(d2); 0 0 0 1]  Output1D=off
  Interpreted MATLAB Function2 : MATLABFcn  MATLABFcn=[cos(u) -sin(u) 0 L2; -sin(u) -cos(u) 0 0; 0 0 -1 0; 0 0 0 1]  Output1D=off
  Product : Product  Inputs=3  Multiplication=Matrix(*)
  Out1 : Outport
  wires:
  Demux1/1 -> Interpreted MATLAB Function/1
  In1/1 -> Demux1/1
  Product/1 -> Out1/1
  Demux1/2 -> Interpreted MATLAB Function1/1
  Demux1/3 -> Interpreted MATLAB Function2/1
  Interpreted MATLAB Function/1 -> Product/1
  Interpreted MATLAB Function1/1 -> Product/2
  Interpreted MATLAB Function2/1 -> Product/3

== system fkine_test1/fkine_R3/fkine_R3_original/T30 ==
  In1 : Inport
  Demux1 : Demux  Outputs=3
  Interpreted MATLAB Function : MATLABFcn  MATLABFcn=[cos(u) -sin(u) 0 0; sin(u) cos(u) 0 0; 0 0 1 d1; 0 0 0 1]  Output1D=off
  Interpreted MATLAB Function1 : MATLABFcn  MATLABFcn=[cos(u) -sin(u) 0 L1; 0 0 -1 0; sin(u) cos(u) 0 -abs(d2); 0 0 0 1]  Output1D=off
  Interpreted MATLAB Function2 : MATLABFcn  MATLABFcn=[cos(u) -sin(u) 0 L2; -sin(u) -cos(u) 0 0; 0 0 -1 0; 0 0 0 1]  Output1D=off
  Product : Product  Inputs=3  Multiplication=Matrix(*)
  Out1 : Outport
  wires:
  Demux1/1 -> Interpreted MATLAB Function/1
  In1/1 -> Demux1/1
  Product/1 -> Out1/1
  Demux1/2 -> Interpreted MATLAB Function1/1
  Demux1/3 -> Interpreted MATLAB Function2/1
  Interpreted MATLAB Function/1 -> Product/1
  Interpreted MATLAB Function1/1 -> Product/2
  Interpreted MATLAB Function2/1 -> Product/3
